simulink model "feixianxing"  (R2019b)
settings: Solver=VariableStepAuto  StartTime=0.0  StopTime=5  MaxStep=0.001  RelTol=1e-3
undefined symbols (not defined in the file): K, T
settings Model: Creator=Inspiron  LastModifiedBy=Inspiron

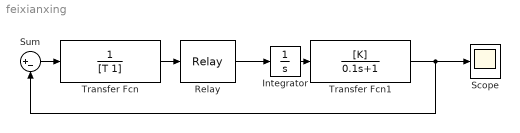
== system feixianxing ==
  Integrator : Integrator
  Relay : Relay  OnSwitchValue=0  OffSwitchValue=0  OnOutputValue=sqrt(2)  OffOutputValue=-sqrt(2)
  Scope : Scope
  Sum : Sum  Inputs=|+-
  Transfer Fcn : TransferFcn  Denominator=[T 1]
  Transfer Fcn1 : TransferFcn  Numerator=[K]  Denominator=[0.1 1]
  wires:
  Transfer Fcn/1 -> Relay/1
  Relay/1 -> Integrator/1
  Integrator/1 -> Transfer Fcn1/1
  Transfer Fcn1/1 -> Scope/1, Sum/2
  Sum/1 -> Transfer Fcn/1
